simulink model "gtm_aeromodel"  (Simulink 7.2)
settings: Solver=ode45  StartTime=0.0  StopTime=10.0  RelTol=1e-3
undefined symbols (not defined in the file or in its folder): A_BLCG, A_BW, A_CW, A_FSCG, A_FSREF_in, A_SW, A_WLCG, A_WLREF, ALPHA0, bclowb, bclowbx_FMACH, bcmowb, bcmowbx_FHP, bcmowby_FMACH, cda, cdax_FLPDEF, cddr, cddrx_FMACH, cdo, cdox_FLPDEF, cdt1, cdt1x_mach, cdt2, cdt2x_mach, cdto, cdtox_mach, cdwb, cdwbx_FALPHA, cdwby_FMACH, clat, clatfr, clatfrx_FHP, clatfry_FMACH, clatx_mach, clawbfr, clawbfrx_FHP, clawbfry_FMACH, cldefr, cldefrx_FHP, cldefry_FMACH, cldtab, cldtabx_FMACH, clqwb, clqwbfr, clqwbfrx_FHP, clqwbfry_FMACH, clqwbx_mach, cltdd, cltddx_FHP, cltddy_FMACH, clwb, clwbtdd, clwbtddx_FHP, clwbtddy_FMACH, clwbx_FALPHA, clwby_FMACH, clwbzdd, clwbzddx_FHP, clwbzddy_FMACH, clzdd ... (+196)
libraries: model_lib x1
(part 9 of 10)

== system gtm_aeromodel/get aero forces and moments/AERODYNAMICS/Moment Coefficients/PITCH/CMWB/CMWBFLEX ==
  note: tddco2g=fqadot*fcbar/(2*32.174)
  altitude : Inport  OutDataType=sfix(16)  OutScaling=2^0
  Mach : Inport  Port=2  OutDataType=sfix(16)  OutScaling=2^0
  NZB g's : Inport  Port=3  OutDataType=sfix(16)  OutScaling=2^0
  qdot : Inport  Port=4  OutDataType=sfix(16)  OutScaling=2^0
  Enable : EnablePort
  Fcn1 : Fcn  Expr=1/u
  Product1 : Product  OutDataType=sfix(16)  OutScaling=2^0  SaturateOnIntegerOverflow=on  RndMeth=Zero  InputSameDT=on  OutDataTypeStr=Inherit: Same as first input
  Product2 : Product  Inputs=3  OutDataType=sfix(16)  OutScaling=2^0  SaturateOnIntegerOverflow=on  RndMeth=Zero  InputSameDT=on  OutDataTypeStr=Inherit: Same as first input
  Product3 : Product  OutDataType=sfix(16)  OutScaling=2^0  SaturateOnIntegerOverflow=on  RndMeth=Zero  InputSameDT=on  OutDataTypeStr=Inherit: Same as first input
  Product4 : Product  OutDataType=sfix(16)  OutScaling=2^0  SaturateOnIntegerOverflow=on  RndMeth=Zero  InputSameDT=on  OutDataTypeStr=Inherit: Same as first input
  Sum3 : Sum  OutDataType=sfix(16)  OutScaling=2^0  SaturateOnIntegerOverflow=on  InputSameDT=on  OutDataTypeStr=Inherit: Same as first input
  Wing Chord : Constant  Value=A_CW  OutDataType=sfix(16)  OutScaling=2^0
  Wing Chord1 : Constant  Value=2  OutDataType=sfix(16)  OutScaling=2^0
  Wing Chord2 : Constant  Value=constants.g  OutDataType=sfix(16)  OutScaling=2^0
  cmawbfr_ : Subsystem  mask(2-D Table){y=cmawbfrx_FHP, z=cmawbfry_FMACH, tab=cmawbfr}
      mask prompts: y "Y vector:"; z "Z vector:"; tab "Table:"
      mask help: 2-D Table Look Up. Enter monotonic Y and Z vectors and a matrix of 2-D tables. See the help for more info.
      mask Help: The Y and Z vectors must be monotonic.  Y  indexes into the columns of the 2-D table & Z indexes into the rows of the 2-D tables.   The input values are y and z respectively (e.g., top port = y).
      mask Display: plot(-10,-10,110,110,[90,50,10],[90,40,30],[90,50,10],[50,26,20],[90,50,10],[22,13,10])
  cmwbtdd : Subsystem  mask(2-D Table){y=cmwbtddx_FHP, z=cmwbtddy_FMACH, tab=cmwbtdd}
      mask prompts: y "Y vector:"; z "Z vector:"; tab "Table:"
      mask help: 2-D Table Look Up. Enter monotonic Y and Z vectors and a matrix of 2-D tables. See the help for more info.
      mask Help: The Y and Z vectors must be monotonic.  Y  indexes into the columns of the 2-D table & Z indexes into the rows of the 2-D tables.   The input values are y and z respectively (e.g., top port = y).
      mask Display: plot(-10,-10,110,110,[90,50,10],[90,40,30],[90,50,10],[50,26,20],[90,50,10],[22,13,10])
  cmwbzdd : Subsystem  mask(2-D Table){y=cmwbzddx_FHP, z=cmwbzddy_FMACH, tab=cmwbzdd}
      mask prompts: y "Y vector:"; z "Z vector:"; tab "Table:"
      mask help: 2-D Table Look Up. Enter monotonic Y and Z vectors and a matrix of 2-D tables. See the help for more info.
      mask Help: The Y and Z vectors must be monotonic.  Y  indexes into the columns of the 2-D table & Z indexes into the rows of the 2-D tables.   The input values are y and z respectively (e.g., top port = y).
      mask Display: plot(-10,-10,110,110,[90,50,10],[90,40,30],[90,50,10],[50,26,20],[90,50,10],[22,13,10])
  dcmowbflex_ : Subsystem  mask(2-D Table){y=dcmowbflexx_FHP, z=dcmowbflexy_FMACH, tab=dcmowbflex}
      mask prompts: y "Y vector:"; z "Z vector:"; tab "Table:"
      mask help: 2-D Table Look Up. Enter monotonic Y and Z vectors and a matrix of 2-D tables. See the help for more info.
      mask Help: The Y and Z vectors must be monotonic.  Y  indexes into the columns of the 2-D table & Z indexes into the rows of the 2-D tables.   The input values are y and z respectively (e.g., top port = y).
      mask Display: plot(-10,-10,110,110,[90,50,10],[90,40,30],[90,50,10],[50,26,20],[90,50,10],[22,13,10])
  cm_flx : Outport  OutDataType=sfix(16)  OutScaling=2^0  InitialOutput=0
  cmawbfr : Outport  Port=2  OutDataType=sfix(16)  OutScaling=2^0  InitialOutput=0
  fdcmowb : Outport  Port=3  OutDataType=sfix(16)  OutScaling=2^0  InitialOutput=0
  wires:
  cmwbzdd/1(Interp Value) -> Product1/1
  cmwbtdd/1(Interp Value) -> Product2/1
  Sum3/1 -> cm_flx/1
  Product1/1 -> Sum3/1
  dcmowbflex_/1(Interp Value) -> fdcmowb/1
  Wing Chord1/1 -> Product4/1
  Fcn1/1 -> Product2/3
  Product3/1 -> Product2/2
  qdot/1 -> Product3/1
  Product4/1 -> Fcn1/1
  Wing Chord2/1 -> Product4/2
  Wing Chord/1 -> Product3/2
  cmawbfr_/1(Interp Value) -> cmawbfr/1
  altitude/1 -> cmwbtdd/1(Y), cmwbzdd/1(Y), cmawbfr_/1(Y), dcmowbflex_/1(Y)
  Mach/1 -> cmwbtdd/2(Z), cmwbzdd/2(Z), cmawbfr_/2(Z), dcmowbflex_/2(Z)
  Product2/1 -> Sum3/2
  NZB g's/1 -> Product1/2

== system gtm_aeromodel/get aero forces and moments/AERODYNAMICS/Moment Coefficients/PITCH/CMWB/cm_flap_ ==
  flap : Inport  OutDataType=sfix(16)  OutScaling=2^0
  alpha : Inport  Port=2  OutDataType=sfix(16)  OutScaling=2^0
  qdyn : Inport  Port=3  OutDataType=sfix(16)  OutScaling=2^0
  flex : Inport  Port=4  OutDataType=sfix(16)  OutScaling=2^0
  dsb : Inport  Port=5  OutDataType=sfix(16)  OutScaling=2^0
  Enable : EnablePort
  DSB : Constant  Value=0.0  OutDataType=sfix(16)  OutScaling=2^0
  MACH : Constant  Value=0.178  OutDataType=sfix(16)  OutScaling=2^0
  Product : Product  OutDataType=sfix(16)  OutScaling=2^0  SaturateOnIntegerOverflow=on  RndMeth=Zero  InputSameDT=on  OutDataTypeStr=Inherit: Same as first input
  Sum : Sum  Inputs=+-  OutDataType=sfix(16)  OutScaling=2^0  SaturateOnIntegerOverflow=on  InputSameDT=on  OutDataTypeStr=Inherit: Same as first input
  Sum1 : Sum  Inputs=+--  OutDataType=sfix(16)  OutScaling=2^0  SaturateOnIntegerOverflow=on  InputSameDT=on  OutDataTypeStr=Inherit: Same as first input
  Switch5 : Switch  Threshold=0.5  SaturateOnIntegerOverflow=on  InputSameDT=on
  cmwb : Subsystem  mask(2-D Table){y=cmwbx_FALPHA, z=cmwby_FMACH, tab=cmwb}
      mask prompts: y "Y vector:"; z "Z vector:"; tab "Table:"
      mask help: 2-D Table Look Up. Enter monotonic Y and Z vectors and a matrix of 2-D tables. See the help for more info.
      mask Help: The Y and Z vectors must be monotonic.  Y  indexes into the columns of the 2-D table & Z indexes into the rows of the 2-D tables.   The input values are y and z respectively (e.g., top port = y).
      mask Display: plot(-10,-10,110,110,[90,50,10],[90,40,30],[90,50,10],[50,26,20],[90,50,10],[22,13,10])
  cmwbdsbdf : Subsystem  mask(1-2-3 Table){@1=cmwbdsbdfx_DSB, @2=cmwbdsbdfy_FALPHA, @3=cmwbdsbdfz_FLPDEF, @4=cmwbdsbdf}
      mask prompts: @1 "X vector:"; @2 "Y vector:"; @3 "Z vector:"; @4 "Table:"
      mask help: 3-D Table Look Up. Enter monotonic X, Y and Z vectors and a matrix of 2-D tables. See the help for more info.
      mask init:
      | x=@1;y=@2;z=@3;tab=@4;
      mask Help: The X, Y and Z vectors must be monotonic.   The 3-D table is a horizontal concatenation of  2-D tables.  X  indexes into the columns of the 2-D tables & Y indexes into the rows of the 2-D tables.  Z indexes into the table levels (starting with the 1st 2-D table).   The input values are x, y and z respectively (e.g., top port = x).
      mask Display: plot([0 2 2 0 0],[0 0 2 2 0],[0 2 2.9 0.95 0],[2 2 2.7 2.7 2],[2 2.9 2.9 2 2],[0 0.85 2.7 2 0])
  cmwbdsbdf1 : Subsystem  mask(1-2-3 Table){@1=cmwbdsbdfx_DSB, @2=cmwbdsbdfy_FALPHA, @3=cmwbdsbdfz_FLPDEF, @4=cmwbdsbdf}
      mask prompts: @1 "X vector:"; @2 "Y vector:"; @3 "Z vector:"; @4 "Table:"
      mask help: 3-D Table Look Up. Enter monotonic X, Y and Z vectors and a matrix of 2-D tables. See the help for more info.
      mask init:
      | x=@1;y=@2;z=@3;tab=@4;
      mask Help: The X, Y and Z vectors must be monotonic.   The 3-D table is a horizontal concatenation of  2-D tables.  X  indexes into the columns of the 2-D tables & Y indexes into the rows of the 2-D tables.  Z indexes into the table levels (starting with the 1st 2-D table).   The input values are x, y and z respectively (e.g., top port = x).
      mask Display: plot([0 2 2 0 0],[0 0 2 2 0],[0 2 2.9 0.95 0],[2 2 2.7 2.7 2],[2 2.9 2.9 2 2],[0 0.85 2.7 2 0])
  const : Constant  Value=1.0  OutDataType=sfix(16)  OutScaling=2^0
  dcmwbdffr : Subsystem  mask(2-D Table){y=dcmwbdffrx_FQ, z=dcmwbdffry_FLPDEF, tab=dcmwbdffr}
      mask prompts: y "Y vector:"; z "Z vector:"; tab "Table:"
      mask help: 2-D Table Look Up. Enter monotonic Y and Z vectors and a matrix of 2-D tables. See the help for more info.
      mask Help: The Y and Z vectors must be monotonic.  Y  indexes into the columns of the 2-D table & Z indexes into the rows of the 2-D tables.   The input values are y and z respectively (e.g., top port = y).
      mask Display: plot(-10,-10,110,110,[90,50,10],[90,40,30],[90,50,10],[50,26,20],[90,50,10],[22,13,10])
  dcmwbdsb : Subsystem  mask(1-2-3 Table){@1=dcmwbdsbx_DSB, @2=dcmwbdsby_ALPHA, @3=dcmwbdsbz_FMACH, @4=dcmwbdsb}
      mask prompts: @1 "X vector:"; @2 "Y vector:"; @3 "Z vector:"; @4 "Table:"
      mask help: 3-D Table Look Up. Enter monotonic X, Y and Z vectors and a matrix of 2-D tables. See the help for more info.
      mask init:
      | x=@1;y=@2;z=@3;tab=@4;
      mask Help: The X, Y and Z vectors must be monotonic.   The 3-D table is a horizontal concatenation of  2-D tables.  X  indexes into the columns of the 2-D tables & Y indexes into the rows of the 2-D tables.  Z indexes into the table levels (starting with the 1st 2-D table).   The input values are x, y and z respectively (e.g., top port = x).
      mask Display: plot([0 2 2 0 0],[0 0 2 2 0],[0 2 2.9 0.95 0],[2 2 2.7 2.7 2],[2 2.9 2.9 2 2],[0 0.85 2.7 2 0])
  cm_flap : Outport  OutDataType=sfix(16)  OutScaling=2^0  InitialOutput=0
  dcmsbfint : Outport  Port=2  OutDataType=sfix(16)  OutScaling=2^0  InitialOutput=0
  wires:
  Sum1/1 -> dcmsbfint/1
  dcmwbdffr/1(Interp Value) -> Switch5/1
  cmwbdsbdf/1(Interp Value) -> Sum1/2, Sum/1
  cmwbdsbdf1/1(Interp Value) -> Sum1/1
  Switch5/1 -> Product/2
  const/1 -> Switch5/3
  flex/1 -> Switch5/2
  qdyn/1 -> dcmwbdffr/1(Y)
  Product/1 -> cm_flap/1
  flap/1 -> cmwbdsbdf1/3(Z), dcmwbdffr/2(Z), cmwbdsbdf/3(Z)
  Sum/1 -> Product/1
  alpha/1 -> cmwbdsbdf/2(Y), cmwbdsbdf1/2(Y), dcmwbdsb/2(Y), cmwb/1(Y)
  DSB/1 -> cmwbdsbdf/1(X)
  dcmwbdsb/1(Interp Value) -> Sum1/3
  MACH/1 -> dcmwbdsb/3(Z), cmwb/2(Z)
  dsb/1 -> cmwbdsbdf1/1(X), dcmwbdsb/1(X)
  cmwb/1(Interp Value) -> Sum/2

== system gtm_aeromodel/get aero forces and moments/AERODYNAMICS/Moment Coefficients/PITCH/CMWB/cmwb_ ==
  Y : Inport  OutDataType=sfix(16)  OutScaling=2^0
  Z : Inport  Port=2  OutDataType=sfix(16)  OutScaling=2^0
  Mux : Mux  Inputs=2
  S-Function : S-Function  FunctionName=table2v5  Parameters=y,z,tab  EnableBusSupport=off
  Interp Value : Outport  OutDataType=sfix(16)  OutScaling=2^0
  wires:
  Mux/1 -> S-Function/1
  S-Function/1 -> Interp Value/1
  Y/1 -> Mux/1
  Z/1 -> Mux/2

== system gtm_aeromodel/get aero forces and moments/AERODYNAMICS/Moment Coefficients/PITCH/CMWB/cmwb_zero ==
  Y : Inport  OutDataType=sfix(16)  OutScaling=2^0
  Z : Inport  Port=2  OutDataType=sfix(16)  OutScaling=2^0
  Mux : Mux  Inputs=2
  S-Function : S-Function  FunctionName=table2v5  Parameters=y,z,tab  EnableBusSupport=off
  Interp Value : Outport  OutDataType=sfix(16)  OutScaling=2^0
  wires:
  Z/1 -> Mux/2
  Y/1 -> Mux/1
  S-Function/1 -> Interp Value/1
  Mux/1 -> S-Function/1

== system gtm_aeromodel/get aero forces and moments/AERODYNAMICS/Moment Coefficients/PITCH/DCMDE/cmdefr ==
  altitude : Inport  OutDataType=sfix(16)  OutScaling=2^0
  mach : Inport  Port=2  OutDataType=sfix(16)  OutScaling=2^0
  Enable : EnablePort
  cmdefr_ : Subsystem  mask(2-D Table){y=cmdefrx_FHP, z=cmdefry_FMACH, tab=cmdefr}
      mask prompts: y "Y vector:"; z "Z vector:"; tab "Table:"
      mask help: 2-D Table Look Up. Enter monotonic Y and Z vectors and a matrix of 2-D tables. See the help for more info.
      mask Help: The Y and Z vectors must be monotonic.  Y  indexes into the columns of the 2-D table & Z indexes into the rows of the 2-D tables.   The input values are y and z respectively (e.g., top port = y).
      mask Display: plot(-10,-10,110,110,[90,50,10],[90,40,30],[90,50,10],[50,26,20],[90,50,10],[22,13,10])
  cmdefr : Outport  OutDataType=sfix(16)  OutScaling=2^0  InitialOutput=0
  wires:
  mach/1 -> cmdefr_/2(Z)
  altitude/1 -> cmdefr_/1(Y)
  cmdefr_/1(Interp Value) -> cmdefr/1

== system gtm_aeromodel/get aero forces and moments/AERODYNAMICS/Moment Coefficients/PITCH/DCMDE/dcmde_ ==
  X : Inport  OutDataType=sfix(16)  OutScaling=2^0
  Y : Inport  Port=2  OutDataType=sfix(16)  OutScaling=2^0
  Z : Inport  Port=3  OutDataType=sfix(16)  OutScaling=2^0
  Mux : Mux  Inputs=3
  S-Function : S-Function  FunctionName=table3v5  Parameters=x,y,z,tab  EnableBusSupport=off
  Interp Value : Outport  OutDataType=sfix(16)  OutScaling=2^0
  wires:
  S-Function/1 -> Interp Value/1
  Mux/1 -> S-Function/1
  X/1 -> Mux/1
  Y/1 -> Mux/2
  Z/1 -> Mux/3

== system gtm_aeromodel/get aero forces and moments/AERODYNAMICS/Moment Coefficients/ROLL/CRAIL/CAILFLEX ==
  altitude : Inport  OutDataType=sfix(16)  OutScaling=2^0
  Mach : Inport  Port=2  OutDataType=sfix(16)  OutScaling=2^0
  Enable : EnablePort
  crdafr_ : Subsystem  mask(2-D Table){y=crdafrx_FHP, z=crdafry_FMACH, tab=crdafr}
      mask prompts: y "Y vector:"; z "Z vector:"; tab "Table:"
      mask help: 2-D Table Look Up. Enter monotonic Y and Z vectors and a matrix of 2-D tables. See the help for more info.
      mask Help: The Y and Z vectors must be monotonic.  Y  indexes into the columns of the 2-D table & Z indexes into the rows of the 2-D tables.   The input values are y and z respectively (e.g., top port = y).
      mask Display: plot(-10,-10,110,110,[90,50,10],[90,40,30],[90,50,10],[50,26,20],[90,50,10],[22,13,10])
  crdafr : Outport  OutDataType=sfix(16)  OutScaling=2^0  InitialOutput=0
  wires:
  altitude/1 -> crdafr_/1(Y)
  Mach/1 -> crdafr_/2(Z)
  crdafr_/1(Interp Value) -> crdafr/1

== system gtm_aeromodel/get aero forces and moments/AERODYNAMICS/Moment Coefficients/ROLL/CRAIL/crda ==
  X : Inport  OutDataType=sfix(16)  OutScaling=2^0
  Y : Inport  Port=2  OutDataType=sfix(16)  OutScaling=2^0
  Z : Inport  Port=3  OutDataType=sfix(16)  OutScaling=2^0
  Mux : Mux  Inputs=3
  S-Function : S-Function  FunctionName=table3v5  Parameters=x,y,z,tab  EnableBusSupport=off
  Interp Value : Outport  OutDataType=sfix(16)  OutScaling=2^0
  wires:
  Z/1 -> Mux/3
  Y/1 -> Mux/2
  X/1 -> Mux/1
  Mux/1 -> S-Function/1
  S-Function/1 -> Interp Value/1

== system gtm_aeromodel/get aero forces and moments/AERODYNAMICS/Moment Coefficients/ROLL/CRAIL/crda1 ==
  X : Inport  OutDataType=sfix(16)  OutScaling=2^0
  Y : Inport  Port=2  OutDataType=sfix(16)  OutScaling=2^0
  Z : Inport  Port=3  OutDataType=sfix(16)  OutScaling=2^0
  Mux : Mux  Inputs=3
  S-Function : S-Function  FunctionName=table3v5  Parameters=x,y,z,tab  EnableBusSupport=off
  Interp Value : Outport  OutDataType=sfix(16)  OutScaling=2^0
  wires:
  S-Function/1 -> Interp Value/1
  Mux/1 -> S-Function/1
  X/1 -> Mux/1
  Y/1 -> Mux/2
  Z/1 -> Mux/3

== system gtm_aeromodel/get aero forces and moments/AERODYNAMICS/Moment Coefficients/ROLL/CRAIL/crdadot ==
  Z : Inport  OutDataType=sfix(16)  OutScaling=2^0
  S-Function : S-Function  FunctionName=table1v5  Parameters=z,tab  EnableBusSupport=off
  Interp Value : Outport  OutDataType=sfix(16)  OutScaling=2^0
  wires:
  S-Function/1 -> Interp Value/1
  Z/1 -> S-Function/1

== system gtm_aeromodel/get aero forces and moments/AERODYNAMICS/Moment Coefficients/ROLL/CRAIL/crdadot1 ==
  Z : Inport  OutDataType=sfix(16)  OutScaling=2^0
  S-Function : S-Function  FunctionName=table1v5  Parameters=z,tab  EnableBusSupport=off
  Interp Value : Outport  OutDataType=sfix(16)  OutScaling=2^0
  wires:
  Z/1 -> S-Function/1
  S-Function/1 -> Interp Value/1

== system gtm_aeromodel/get aero forces and moments/AERODYNAMICS/Moment Coefficients/ROLL/CRBWB/CRWBFLEX ==
  altitude : Inport  OutDataType=sfix(16)  OutScaling=2^0
  Mach : Inport  Port=2  OutDataType=sfix(16)  OutScaling=2^0
  Enable : EnablePort
  crbfr_ : Subsystem  mask(2-D Table){y=crbfrx_FHP, z=crbfry_FMACH, tab=crbfr}
      mask prompts: y "Y vector:"; z "Z vector:"; tab "Table:"
      mask help: 2-D Table Look Up. Enter monotonic Y and Z vectors and a matrix of 2-D tables. See the help for more info.
      mask Help: The Y and Z vectors must be monotonic.  Y  indexes into the columns of the 2-D table & Z indexes into the rows of the 2-D tables.   The input values are y and z respectively (e.g., top port = y).
      mask Display: plot(-10,-10,110,110,[90,50,10],[90,40,30],[90,50,10],[50,26,20],[90,50,10],[22,13,10])
  crbfr : Outport  OutDataType=sfix(16)  OutScaling=2^0  InitialOutput=0
  wires:
  Mach/1 -> crbfr_/2(Z)
  altitude/1 -> crbfr_/1(Y)
  crbfr_/1(Interp Value) -> crbfr/1

== system gtm_aeromodel/get aero forces and moments/AERODYNAMICS/Moment Coefficients/ROLL/CRBWB/cr_flap_ ==
  flap : Inport  OutDataType=sfix(16)  OutScaling=2^0
  alpha : Inport  Port=2  OutDataType=sfix(16)  OutScaling=2^0
  Enable : EnablePort
  dcrbdf1 : Subsystem  mask(2-D Table){y=dcrbdfx_FLPDEF, z=dcrbdfy_FALPHA, tab=dcrbdf}
      mask prompts: y "Y vector:"; z "Z vector:"; tab "Table:"
      mask help: 2-D Table Look Up. Enter monotonic Y and Z vectors and a matrix of 2-D tables. See the help for more info.
      mask Help: The Y and Z vectors must be monotonic.  Y  indexes into the columns of the 2-D table & Z indexes into the rows of the 2-D tables.   The input values are y and z respectively (e.g., top port = y).
      mask Display: plot(-10,-10,110,110,[90,50,10],[90,40,30],[90,50,10],[50,26,20],[90,50,10],[22,13,10])
  cr_flap : Outport  OutDataType=sfix(16)  OutScaling=2^0  InitialOutput=0
  wires:
  flap/1 -> dcrbdf1/1(Y)
  alpha/1 -> dcrbdf1/2(Z)
  dcrbdf1/1(Interp Value) -> cr_flap/1

== system gtm_aeromodel/get aero forces and moments/AERODYNAMICS/Moment Coefficients/ROLL/CRBWB/crbwb_ ==
  Y : Inport  OutDataType=sfix(16)  OutScaling=2^0
  Z : Inport  Port=2  OutDataType=sfix(16)  OutScaling=2^0
  Mux : Mux  Inputs=2
  S-Function : S-Function  FunctionName=table2v5  Parameters=y,z,tab  EnableBusSupport=off
  Interp Value : Outport  OutDataType=sfix(16)  OutScaling=2^0
  wires:
  Z/1 -> Mux/2
  Y/1 -> Mux/1
  S-Function/1 -> Interp Value/1
  Mux/1 -> S-Function/1

== system gtm_aeromodel/get aero forces and moments/AERODYNAMICS/Moment Coefficients/ROLL/CRGEAR/dcrb_ ==
  Z : Inport  OutDataType=sfix(16)  OutScaling=2^0
  S-Function : S-Function  FunctionName=table1v5  Parameters=z,tab  EnableBusSupport=off
  Interp Value : Outport  OutDataType=sfix(16)  OutScaling=2^0
  wires:
  Z/1 -> S-Function/1
  S-Function/1 -> Interp Value/1

== system gtm_aeromodel/get aero forces and moments/AERODYNAMICS/Moment Coefficients/ROLL/CRP/CRPFLEX ==
  altitude : Inport  OutDataType=sfix(16)  OutScaling=2^0
  Mach : Inport  Port=2  OutDataType=sfix(16)  OutScaling=2^0
  Enable : EnablePort
  crpfr_ : Subsystem  mask(2-D Table){y=crpfrx_FHP, z=crpfry_FMACH, tab=crpfr}
      mask prompts: y "Y vector:"; z "Z vector:"; tab "Table:"
      mask help: 2-D Table Look Up. Enter monotonic Y and Z vectors and a matrix of 2-D tables. See the help for more info.
      mask Help: The Y and Z vectors must be monotonic.  Y  indexes into the columns of the 2-D table & Z indexes into the rows of the 2-D tables.   The input values are y and z respectively (e.g., top port = y).
      mask Display: plot(-10,-10,110,110,[90,50,10],[90,40,30],[90,50,10],[50,26,20],[90,50,10],[22,13,10])
  crpfr : Outport  OutDataType=sfix(16)  OutScaling=2^0  InitialOutput=0
  wires:
  Mach/1 -> crpfr_/2(Z)
  altitude/1 -> crpfr_/1(Y)
  crpfr_/1(Interp Value) -> crpfr/1

== system gtm_aeromodel/get aero forces and moments/AERODYNAMICS/Moment Coefficients/ROLL/CRP/crpwb_ ==
  Y : Inport  OutDataType=sfix(16)  OutScaling=2^0
  Z : Inport  Port=2  OutDataType=sfix(16)  OutScaling=2^0
  Mux : Mux  Inputs=2
  S-Function : S-Function  FunctionName=table2v5  Parameters=y,z,tab  EnableBusSupport=off
  Interp Value : Outport  OutDataType=sfix(16)  OutScaling=2^0
  wires:
  Z/1 -> Mux/2
  Y/1 -> Mux/1
  S-Function/1 -> Interp Value/1
  Mux/1 -> S-Function/1

== system gtm_aeromodel/get aero forces and moments/AERODYNAMICS/Moment Coefficients/ROLL/CRP/rcrbvt ==
  Y : Inport  OutDataType=sfix(16)  OutScaling=2^0
  Z : Inport  Port=2  OutDataType=sfix(16)  OutScaling=2^0
  Mux : Mux  Inputs=2
  S-Function : S-Function  FunctionName=table2v5  Parameters=y,z,tab  EnableBusSupport=off
  Interp Value : Outport  OutDataType=sfix(16)  OutScaling=2^0
  wires:
  Mux/1 -> S-Function/1
  S-Function/1 -> Interp Value/1
  Y/1 -> Mux/1
  Z/1 -> Mux/2

== system gtm_aeromodel/get aero forces and moments/AERODYNAMICS/Moment Coefficients/ROLL/CRP/rcybvt ==
  Y : Inport  OutDataType=sfix(16)  OutScaling=2^0
  Z : Inport  Port=2  OutDataType=sfix(16)  OutScaling=2^0
  Mux : Mux  Inputs=2
  S-Function : S-Function  FunctionName=table2v5  Parameters=y,z,tab  EnableBusSupport=off
  Interp Value : Outport  OutDataType=sfix(16)  OutScaling=2^0
  wires:
  Z/1 -> Mux/2
  Y/1 -> Mux/1
  S-Function/1 -> Interp Value/1
  Mux/1 -> S-Function/1

== system gtm_aeromodel/get aero forces and moments/AERODYNAMICS/Moment Coefficients/ROLL/CRR/CRRFLEX ==
  altitude : Inport  OutDataType=sfix(16)  OutScaling=2^0
  Mach : Inport  Port=2  OutDataType=sfix(16)  OutScaling=2^0
  Enable : EnablePort
  crrfr_ : Subsystem  mask(2-D Table){y=crrfrx_FHP, z=crrfry_FMACH, tab=crrfr}
      mask prompts: y "Y vector:"; z "Z vector:"; tab "Table:"
      mask help: 2-D Table Look Up. Enter monotonic Y and Z vectors and a matrix of 2-D tables. See the help for more info.
      mask Help: The Y and Z vectors must be monotonic.  Y  indexes into the columns of the 2-D table & Z indexes into the rows of the 2-D tables.   The input values are y and z respectively (e.g., top port = y).
      mask Display: plot(-10,-10,110,110,[90,50,10],[90,40,30],[90,50,10],[50,26,20],[90,50,10],[22,13,10])
  crrfr : Outport  OutDataType=sfix(16)  OutScaling=2^0  InitialOutput=0
  wires:
  altitude/1 -> crrfr_/1(Y)
  Mach/1 -> crrfr_/2(Z)
  crrfr_/1(Interp Value) -> crrfr/1

== system gtm_aeromodel/get aero forces and moments/AERODYNAMICS/Moment Coefficients/ROLL/CRR/crrwb_ ==
  Y : Inport  OutDataType=sfix(16)  OutScaling=2^0
  Z : Inport  Port=2  OutDataType=sfix(16)  OutScaling=2^0
  Mux : Mux  Inputs=2
  S-Function : S-Function  FunctionName=table2v5  Parameters=y,z,tab  EnableBusSupport=off
  Interp Value : Outport  OutDataType=sfix(16)  OutScaling=2^0
  wires:
  Z/1 -> Mux/2
  Y/1 -> Mux/1
  S-Function/1 -> Interp Value/1
  Mux/1 -> S-Function/1

== system gtm_aeromodel/get aero forces and moments/AERODYNAMICS/Moment Coefficients/ROLL/CRR/rcnbvt ==
  Y : Inport  OutDataType=sfix(16)  OutScaling=2^0
  Z : Inport  Port=2  OutDataType=sfix(16)  OutScaling=2^0
  Mux : Mux  Inputs=2
  S-Function : S-Function  FunctionName=table2v5  Parameters=y,z,tab  EnableBusSupport=off
  Interp Value : Outport  OutDataType=sfix(16)  OutScaling=2^0
  wires:
  Mux/1 -> S-Function/1
  S-Function/1 -> Interp Value/1
  Y/1 -> Mux/1
  Z/1 -> Mux/2

== system gtm_aeromodel/get aero forces and moments/AERODYNAMICS/Moment Coefficients/ROLL/CRR/rcrbvt ==
  Y : Inport  OutDataType=sfix(16)  OutScaling=2^0
  Z : Inport  Port=2  OutDataType=sfix(16)  OutScaling=2^0
  Mux : Mux  Inputs=2
  S-Function : S-Function  FunctionName=table2v5  Parameters=y,z,tab  EnableBusSupport=off
  Interp Value : Outport  OutDataType=sfix(16)  OutScaling=2^0
  wires:
  Mux/1 -> S-Function/1
  S-Function/1 -> Interp Value/1
  Y/1 -> Mux/1
  Z/1 -> Mux/2

== system gtm_aeromodel/get aero forces and moments/AERODYNAMICS/Moment Coefficients/ROLL/CRR/rcybvt ==
  Y : Inport  OutDataType=sfix(16)  OutScaling=2^0
  Z : Inport  Port=2  OutDataType=sfix(16)  OutScaling=2^0
  Mux : Mux  Inputs=2
  S-Function : S-Function  FunctionName=table2v5  Parameters=y,z,tab  EnableBusSupport=off
  Interp Value : Outport  OutDataType=sfix(16)  OutScaling=2^0
  wires:
  Z/1 -> Mux/2
  Y/1 -> Mux/1
  S-Function/1 -> Interp Value/1
  Mux/1 -> S-Function/1

== system gtm_aeromodel/get aero forces and moments/AERODYNAMICS/Moment Coefficients/ROLL/CRRUD/CRFLEX ==
  altitude : Inport  OutDataType=sfix(16)  OutScaling=2^0
  Mach : Inport  Port=2  OutDataType=sfix(16)  OutScaling=2^0
  Enable : EnablePort
  crdrfr2 : Subsystem  mask(2-D Table){y=crdrfrx_FHP, z=crdrfry_FMACH, tab=crdrfr}
      mask prompts: y "Y vector:"; z "Z vector:"; tab "Table:"
      mask help: 2-D Table Look Up. Enter monotonic Y and Z vectors and a matrix of 2-D tables. See the help for more info.
      mask Help: The Y and Z vectors must be monotonic.  Y  indexes into the columns of the 2-D table & Z indexes into the rows of the 2-D tables.   The input values are y and z respectively (e.g., top port = y).
      mask Display: plot(-10,-10,110,110,[90,50,10],[90,40,30],[90,50,10],[50,26,20],[90,50,10],[22,13,10])
  crdrfr : Outport  OutDataType=sfix(16)  OutScaling=2^0  InitialOutput=0
  wires:
  crdrfr2/1(Interp Value) -> crdrfr/1
  altitude/1 -> crdrfr2/1(Y)
  Mach/1 -> crdrfr2/2(Z)

== system gtm_aeromodel/get aero forces and moments/AERODYNAMICS/Moment Coefficients/ROLL/CRRUD/crdr ==
  Z : Inport  OutDataType=sfix(16)  OutScaling=2^0
  S-Function : S-Function  FunctionName=table1v5  Parameters=z,tab  EnableBusSupport=off
  Interp Value : Outport  OutDataType=sfix(16)  OutScaling=2^0
  wires:
  S-Function/1 -> Interp Value/1
  Z/1 -> S-Function/1

== system gtm_aeromodel/get aero forces and moments/AERODYNAMICS/Moment Coefficients/ROLL/CRSPOIL/cr_sp_fl ==
  flap : Inport  OutDataType=sfix(16)  OutScaling=2^0
  alpha : Inport  Port=2  OutDataType=sfix(16)  OutScaling=2^0
  dsl : Inport  Port=3  OutDataType=sfix(16)  OutScaling=2^0
  dsb : Inport  Port=4  OutDataType=sfix(16)  OutScaling=2^0
  dsr : Inport  Port=5  OutDataType=sfix(16)  OutScaling=2^0
  Enable : EnablePort
  Sum1 : Sum  Inputs=+-  OutDataType=sfix(16)  OutScaling=2^0  SaturateOnIntegerOverflow=on  InputSameDT=on  OutDataTypeStr=Inherit: Same as first input
  Sum2 : Sum  Inputs=+-  OutDataType=sfix(16)  OutScaling=2^0  SaturateOnIntegerOverflow=on  InputSameDT=on  OutDataTypeStr=Inherit: Same as first input
  Sum3 : Sum  Inputs=+-  OutDataType=sfix(16)  OutScaling=2^0  SaturateOnIntegerOverflow=on  InputSameDT=on  OutDataTypeStr=Inherit: Same as first input
  dcrwbdsldf : Subsystem  mask(1-2-3 Table){@1=dcrwbdsldfx_DSL, @2=dcrwbdsldfy_FALPHA, @3=dcrwbdsldfz_FLPDEF, @4=dcrwbdsldf}
      mask prompts: @1 "X vector:"; @2 "Y vector:"; @3 "Z vector:"; @4 "Table:"
      mask help: 3-D Table Look Up. Enter monotonic X, Y and Z vectors and a matrix of 2-D tables. See the help for more info.
      mask init:
      | x=@1;y=@2;z=@3;tab=@4;
      mask Help: The X, Y and Z vectors must be monotonic.   The 3-D table is a horizontal concatenation of  2-D tables.  X  indexes into the columns of the 2-D tables & Y indexes into the rows of the 2-D tables.  Z indexes into the table levels (starting with the 1st 2-D table).   The input values are x, y and z respectively (e.g., top port = x).
      mask Display: plot([0 2 2 0 0],[0 0 2 2 0],[0 2 2.9 0.95 0],[2 2 2.7 2.7 2],[2 2.9 2.9 2 2],[0 0.85 2.7 2 0])
  dcrwbdsldf1 : Subsystem  mask(1-2-3 Table){@1=dcrwbdsldfx_DSL, @2=dcrwbdsldfy_FALPHA, @3=dcrwbdsldfz_FLPDEF, @4=dcrwbdsldf}
      mask prompts: @1 "X vector:"; @2 "Y vector:"; @3 "Z vector:"; @4 "Table:"
      mask help: 3-D Table Look Up. Enter monotonic X, Y and Z vectors and a matrix of 2-D tables. See the help for more info.
      mask init:
      | x=@1;y=@2;z=@3;tab=@4;
      mask Help: The X, Y and Z vectors must be monotonic.   The 3-D table is a horizontal concatenation of  2-D tables.  X  indexes into the columns of the 2-D tables & Y indexes into the rows of the 2-D tables.  Z indexes into the table levels (starting with the 1st 2-D table).   The input values are x, y and z respectively (e.g., top port = x).
      mask Display: plot([0 2 2 0 0],[0 0 2 2 0],[0 2 2.9 0.95 0],[2 2 2.7 2.7 2],[2 2.9 2.9 2 2],[0 0.85 2.7 2 0])
  dcrwbdsldf2 : Subsystem  mask(1-2-3 Table){@1=dcrwbdsldfx_DSL, @2=dcrwbdsldfy_FALPHA, @3=dcrwbdsldfz_FLPDEF, @4=dcrwbdsldf}
      mask prompts: @1 "X vector:"; @2 "Y vector:"; @3 "Z vector:"; @4 "Table:"
      mask help: 3-D Table Look Up. Enter monotonic X, Y and Z vectors and a matrix of 2-D tables. See the help for more info.
      mask init:
      | x=@1;y=@2;z=@3;tab=@4;
      mask Help: The X, Y and Z vectors must be monotonic.   The 3-D table is a horizontal concatenation of  2-D tables.  X  indexes into the columns of the 2-D tables & Y indexes into the rows of the 2-D tables.  Z indexes into the table levels (starting with the 1st 2-D table).   The input values are x, y and z respectively (e.g., top port = x).
      mask Display: plot([0 2 2 0 0],[0 0 2 2 0],[0 2 2.9 0.95 0],[2 2 2.7 2.7 2],[2 2.9 2.9 2 2],[0 0.85 2.7 2 0])
  cr_sp_fl : Outport  OutDataType=sfix(16)  OutScaling=2^0  InitialOutput=0
  wires:
  alpha/1 -> dcrwbdsldf/2(Y), dcrwbdsldf1/2(Y), dcrwbdsldf2/2(Y)
  dsl/1 -> dcrwbdsldf/1(X)
  dsb/1 -> dcrwbdsldf1/1(X)
  flap/1 -> dcrwbdsldf/3(Z), dcrwbdsldf1/3(Z), dcrwbdsldf2/3(Z)
  dcrwbdsldf/1(Interp Value) -> Sum1/1
  dsr/1 -> dcrwbdsldf2/1(X)
  dcrwbdsldf2/1(Interp Value) -> Sum2/1
  dcrwbdsldf1/1(Interp Value) -> Sum1/2, Sum2/2
  Sum1/1 -> Sum3/1
  Sum2/1 -> Sum3/2
  Sum3/1 -> cr_sp_fl/1

== system gtm_aeromodel/get aero forces and moments/AERODYNAMICS/Moment Coefficients/ROLL/CRSPOIL/cr_sp_flex ==
  altitude : Inport  OutDataType=sfix(16)  OutScaling=2^0
  mach : Inport  Port=2  OutDataType=sfix(16)  OutScaling=2^0
  Enable : EnablePort
  dcrdslfr : Subsystem  mask(2-D Table){y=dcrdslfrx_FHP, z=dcrdslfry_FMACH, tab=dcrdslfr}
      mask prompts: y "Y vector:"; z "Z vector:"; tab "Table:"
      mask help: 2-D Table Look Up. Enter monotonic Y and Z vectors and a matrix of 2-D tables. See the help for more info.
      mask Help: The Y and Z vectors must be monotonic.  Y  indexes into the columns of the 2-D table & Z indexes into the rows of the 2-D tables.   The input values are y and z respectively (e.g., top port = y).
      mask Display: plot(-10,-10,110,110,[90,50,10],[90,40,30],[90,50,10],[50,26,20],[90,50,10],[22,13,10])
  cr_sp_flex : Outport  OutDataType=sfix(16)  OutScaling=2^0  InitialOutput=0
  wires:
  dcrdslfr/1(Interp Value) -> cr_sp_flex/1
  mach/1 -> dcrdslfr/2(Z)
  altitude/1 -> dcrdslfr/1(Y)

== system gtm_aeromodel/get aero forces and moments/AERODYNAMICS/Moment Coefficients/ROLL/CRSPOIL/dcrwbdsbp ==
  X : Inport  OutDataType=sfix(16)  OutScaling=2^0
  Y : Inport  Port=2  OutDataType=sfix(16)  OutScaling=2^0
  Z : Inport  Port=3  OutDataType=sfix(16)  OutScaling=2^0
  Mux : Mux  Inputs=3
  S-Function : S-Function  FunctionName=table3v5  Parameters=x,y,z,tab  EnableBusSupport=off
  Interp Value : Outport  OutDataType=sfix(16)  OutScaling=2^0
  wires:
  Z/1 -> Mux/3
  Y/1 -> Mux/2
  X/1 -> Mux/1
  Mux/1 -> S-Function/1
  S-Function/1 -> Interp Value/1

== system gtm_aeromodel/get aero forces and moments/AERODYNAMICS/Moment Coefficients/ROLL/CRSPOIL/dcrwbdsl ==
  X : Inport  OutDataType=sfix(16)  OutScaling=2^0
  Y : Inport  Port=2  OutDataType=sfix(16)  OutScaling=2^0
  Z : Inport  Port=3  OutDataType=sfix(16)  OutScaling=2^0
  Mux : Mux  Inputs=3
  S-Function : S-Function  FunctionName=table3v5  Parameters=x,y,z,tab  EnableBusSupport=off
  Interp Value : Outport  OutDataType=sfix(16)  OutScaling=2^0
  wires:
  S-Function/1 -> Interp Value/1
  Mux/1 -> S-Function/1
  X/1 -> Mux/1
  Y/1 -> Mux/2
  Z/1 -> Mux/3

== system gtm_aeromodel/get aero forces and moments/AERODYNAMICS/Moment Coefficients/ROLL/CRSPOIL/dcrwbdsl1 ==
  X : Inport  OutDataType=sfix(16)  OutScaling=2^0
  Y : Inport  Port=2  OutDataType=sfix(16)  OutScaling=2^0
  Z : Inport  Port=3  OutDataType=sfix(16)  OutScaling=2^0
  Mux : Mux  Inputs=3
  S-Function : S-Function  FunctionName=table3v5  Parameters=x,y,z,tab  EnableBusSupport=off
  Interp Value : Outport  OutDataType=sfix(16)  OutScaling=2^0
  wires:
  Z/1 -> Mux/3
  Y/1 -> Mux/2
  X/1 -> Mux/1
  Mux/1 -> S-Function/1
  S-Function/1 -> Interp Value/1

== system gtm_aeromodel/get aero forces and moments/AERODYNAMICS/Moment Coefficients/ROLL/CRSPOIL/dcrwbdsl2 ==
  X : Inport  OutDataType=sfix(16)  OutScaling=2^0
  Y : Inport  Port=2  OutDataType=sfix(16)  OutScaling=2^0
  Z : Inport  Port=3  OutDataType=sfix(16)  OutScaling=2^0
  Mux : Mux  Inputs=3
  S-Function : S-Function  FunctionName=table3v5  Parameters=x,y,z,tab  EnableBusSupport=off
  Interp Value : Outport  OutDataType=sfix(16)  OutScaling=2^0
  wires:
  S-Function/1 -> Interp Value/1
  Mux/1 -> S-Function/1
  X/1 -> Mux/1
  Y/1 -> Mux/2
  Z/1 -> Mux/3

== system gtm_aeromodel/get aero forces and moments/AERODYNAMICS/Moment Coefficients/ROLL/CRSPOIL/dcrwbdsl3 ==
  X : Inport  OutDataType=sfix(16)  OutScaling=2^0
  Y : Inport  Port=2  OutDataType=sfix(16)  OutScaling=2^0
  Z : Inport  Port=3  OutDataType=sfix(16)  OutScaling=2^0
  Mux : Mux  Inputs=3
  S-Function : S-Function  FunctionName=table3v5  Parameters=x,y,z,tab  EnableBusSupport=off
  Interp Value : Outport  OutDataType=sfix(16)  OutScaling=2^0
  wires:
  Z/1 -> Mux/3
  Y/1 -> Mux/2
  X/1 -> Mux/1
  Mux/1 -> S-Function/1
  S-Function/1 -> Interp Value/1

== system gtm_aeromodel/get aero forces and moments/AERODYNAMICS/Moment Coefficients/ROLL/CRSPOIL/dcrwbdsl4 ==
  X : Inport  OutDataType=sfix(16)  OutScaling=2^0
  Y : Inport  Port=2  OutDataType=sfix(16)  OutScaling=2^0
  Z : Inport  Port=3  OutDataType=sfix(16)  OutScaling=2^0
  Mux : Mux  Inputs=3
  S-Function : S-Function  FunctionName=table3v5  Parameters=x,y,z,tab  EnableBusSupport=off
  Interp Value : Outport  OutDataType=sfix(16)  OutScaling=2^0
  wires:
  S-Function/1 -> Interp Value/1
  Mux/1 -> S-Function/1
  X/1 -> Mux/1
  Y/1 -> Mux/2
  Z/1 -> Mux/3

== system gtm_aeromodel/get aero forces and moments/AERODYNAMICS/Moment Coefficients/ROLL/TAIL/crbht ==
  Y : Inport  OutDataType=sfix(16)  OutScaling=2^0
  Z : Inport  Port=2  OutDataType=sfix(16)  OutScaling=2^0
  Mux : Mux  Inputs=2
  S-Function : S-Function  FunctionName=table2v5  Parameters=y,z,tab  EnableBusSupport=off
  Interp Value : Outport  OutDataType=sfix(16)  OutScaling=2^0
  wires:
  Z/1 -> Mux/2
  Y/1 -> Mux/1
  S-Function/1 -> Interp Value/1
  Mux/1 -> S-Function/1

== system gtm_aeromodel/get aero forces and moments/AERODYNAMICS/Moment Coefficients/ROLL/TAIL/crbvt ==
  Y : Inport  OutDataType=sfix(16)  OutScaling=2^0
  Z : Inport  Port=2  OutDataType=sfix(16)  OutScaling=2^0
  Mux : Mux  Inputs=2
  S-Function : S-Function  FunctionName=table2v5  Parameters=y,z,tab  EnableBusSupport=off
  Interp Value : Outport  OutDataType=sfix(16)  OutScaling=2^0
  wires:
  Z/1 -> Mux/2
  Y/1 -> Mux/1
  S-Function/1 -> Interp Value/1
  Mux/1 -> S-Function/1

== system gtm_aeromodel/get aero forces and moments/AERODYNAMICS/Moment Coefficients/YAW/CNBWB/CNWBFLEX ==
  altitude : Inport  OutDataType=sfix(16)  OutScaling=2^0
  Mach : Inport  Port=2  OutDataType=sfix(16)  OutScaling=2^0
  Enable : EnablePort
  cnbfr_ : Subsystem  mask(2-D Table){y=cnbfrx_FHP, z=cnbfry_FMACH, tab=cnbfr}
      mask prompts: y "Y vector:"; z "Z vector:"; tab "Table:"
      mask help: 2-D Table Look Up. Enter monotonic Y and Z vectors and a matrix of 2-D tables. See the help for more info.
      mask Help: The Y and Z vectors must be monotonic.  Y  indexes into the columns of the 2-D table & Z indexes into the rows of the 2-D tables.   The input values are y and z respectively (e.g., top port = y).
      mask Display: plot(-10,-10,110,110,[90,50,10],[90,40,30],[90,50,10],[50,26,20],[90,50,10],[22,13,10])
  cnbfr : Outport  OutDataType=sfix(16)  OutScaling=2^0  InitialOutput=0
  wires:
  cnbfr_/1(Interp Value) -> cnbfr/1
  altitude/1 -> cnbfr_/1(Y)
  Mach/1 -> cnbfr_/2(Z)

== system gtm_aeromodel/get aero forces and moments/AERODYNAMICS/Moment Coefficients/YAW/CNBWB/cn_flap_ ==
  flap : Inport  OutDataType=sfix(16)  OutScaling=2^0
  alpha : Inport  Port=2  OutDataType=sfix(16)  OutScaling=2^0
  Enable : EnablePort
  dcnbdf : Subsystem  mask(2-D Table){y=dcnbdfx_FLPDEF, z=dcnbdfy_FALPHA, tab=dcnbdf}
      mask prompts: y "Y vector:"; z "Z vector:"; tab "Table:"
      mask help: 2-D Table Look Up. Enter monotonic Y and Z vectors and a matrix of 2-D tables. See the help for more info.
      mask Help: The Y and Z vectors must be monotonic.  Y  indexes into the columns of the 2-D table & Z indexes into the rows of the 2-D tables.   The input values are y and z respectively (e.g., top port = y).
      mask Display: plot(-10,-10,110,110,[90,50,10],[90,40,30],[90,50,10],[50,26,20],[90,50,10],[22,13,10])
  cn_flap : Outport  OutDataType=sfix(16)  OutScaling=2^0  InitialOutput=0
  wires:
  alpha/1 -> dcnbdf/2(Z)
  flap/1 -> dcnbdf/1(Y)
  dcnbdf/1(Interp Value) -> cn_flap/1

== system gtm_aeromodel/get aero forces and moments/AERODYNAMICS/Moment Coefficients/YAW/CNBWB/cnbwb_ ==
  Y : Inport  OutDataType=sfix(16)  OutScaling=2^0
  Z : Inport  Port=2  OutDataType=sfix(16)  OutScaling=2^0
  Mux : Mux  Inputs=2
  S-Function : S-Function  FunctionName=table2v5  Parameters=y,z,tab  EnableBusSupport=off
  Interp Value : Outport  OutDataType=sfix(16)  OutScaling=2^0
  wires:
  Z/1 -> Mux/2
  Y/1 -> Mux/1
  S-Function/1 -> Interp Value/1
  Mux/1 -> S-Function/1

== system gtm_aeromodel/get aero forces and moments/AERODYNAMICS/Moment Coefficients/YAW/CNGEAR/dcnb ==
  Z : Inport  OutDataType=sfix(16)  OutScaling=2^0
  S-Function : S-Function  FunctionName=table1v5  Parameters=z,tab  EnableBusSupport=off
  Interp Value : Outport  OutDataType=sfix(16)  OutScaling=2^0
  wires:
  S-Function/1 -> Interp Value/1
  Z/1 -> S-Function/1

== system gtm_aeromodel/get aero forces and moments/AERODYNAMICS/Moment Coefficients/YAW/CNP/CNPFLEX ==
  altitude : Inport  OutDataType=sfix(16)  OutScaling=2^0
  Mach : Inport  Port=2  OutDataType=sfix(16)  OutScaling=2^0
  Enable : EnablePort
  cnpfr_ : Subsystem  mask(2-D Table){y=cnpfrx_FHP, z=cnpfry_FMACH, tab=cnpfr}
      mask prompts: y "Y vector:"; z "Z vector:"; tab "Table:"
      mask help: 2-D Table Look Up. Enter monotonic Y and Z vectors and a matrix of 2-D tables. See the help for more info.
      mask Help: The Y and Z vectors must be monotonic.  Y  indexes into the columns of the 2-D table & Z indexes into the rows of the 2-D tables.   The input values are y and z respectively (e.g., top port = y).
      mask Display: plot(-10,-10,110,110,[90,50,10],[90,40,30],[90,50,10],[50,26,20],[90,50,10],[22,13,10])
  cnpfr : Outport  OutDataType=sfix(16)  OutScaling=2^0  InitialOutput=0
  wires:
  altitude/1 -> cnpfr_/1(Y)
  Mach/1 -> cnpfr_/2(Z)
  cnpfr_/1(Interp Value) -> cnpfr/1

== system gtm_aeromodel/get aero forces and moments/AERODYNAMICS/Moment Coefficients/YAW/CNP/rcnbvt ==
  Y : Inport  OutDataType=sfix(16)  OutScaling=2^0
  Z : Inport  Port=2  OutDataType=sfix(16)  OutScaling=2^0
  Mux : Mux  Inputs=2
  S-Function : S-Function  FunctionName=table2v5  Parameters=y,z,tab  EnableBusSupport=off
  Interp Value : Outport  OutDataType=sfix(16)  OutScaling=2^0
  wires:
  Z/1 -> Mux/2
  Y/1 -> Mux/1
  S-Function/1 -> Interp Value/1
  Mux/1 -> S-Function/1

== system gtm_aeromodel/get aero forces and moments/AERODYNAMICS/Moment Coefficients/YAW/CNP/rcnpwb ==
  Y : Inport  OutDataType=sfix(16)  OutScaling=2^0
  Z : Inport  Port=2  OutDataType=sfix(16)  OutScaling=2^0
  Mux : Mux  Inputs=2
  S-Function : S-Function  FunctionName=table2v5  Parameters=y,z,tab  EnableBusSupport=off
  Interp Value : Outport  OutDataType=sfix(16)  OutScaling=2^0
  wires:
  Z/1 -> Mux/2
  Y/1 -> Mux/1
  S-Function/1 -> Interp Value/1
  Mux/1 -> S-Function/1

== system gtm_aeromodel/get aero forces and moments/AERODYNAMICS/Moment Coefficients/YAW/CNP/rcrbvt ==
  Y : Inport  OutDataType=sfix(16)  OutScaling=2^0
  Z : Inport  Port=2  OutDataType=sfix(16)  OutScaling=2^0
  Mux : Mux  Inputs=2
  S-Function : S-Function  FunctionName=table2v5  Parameters=y,z,tab  EnableBusSupport=off
  Interp Value : Outport  OutDataType=sfix(16)  OutScaling=2^0
  wires:
  Z/1 -> Mux/2
  Y/1 -> Mux/1
  S-Function/1 -> Interp Value/1
  Mux/1 -> S-Function/1

== system gtm_aeromodel/get aero forces and moments/AERODYNAMICS/Moment Coefficients/YAW/CNP/rcybvt ==
  Y : Inport  OutDataType=sfix(16)  OutScaling=2^0
  Z : Inport  Port=2  OutDataType=sfix(16)  OutScaling=2^0
  Mux : Mux  Inputs=2
  S-Function : S-Function  FunctionName=table2v5  Parameters=y,z,tab  EnableBusSupport=off
  Interp Value : Outport  OutDataType=sfix(16)  OutScaling=2^0
  wires:
  Mux/1 -> S-Function/1
  S-Function/1 -> Interp Value/1
  Y/1 -> Mux/1
  Z/1 -> Mux/2

== system gtm_aeromodel/get aero forces and moments/AERODYNAMICS/Moment Coefficients/YAW/CNR/CNRFLEX ==
  altitude : Inport  OutDataType=sfix(16)  OutScaling=2^0
  Mach : Inport  Port=2  OutDataType=sfix(16)  OutScaling=2^0
  Enable : EnablePort
  cnrfr_ : Subsystem  mask(2-D Table){y=cnrfrx_FHP, z=cnrfry_FMACH, tab=cnrfr}
      mask prompts: y "Y vector:"; z "Z vector:"; tab "Table:"
      mask help: 2-D Table Look Up. Enter monotonic Y and Z vectors and a matrix of 2-D tables. See the help for more info.
      mask Help: The Y and Z vectors must be monotonic.  Y  indexes into the columns of the 2-D table & Z indexes into the rows of the 2-D tables.   The input values are y and z respectively (e.g., top port = y).
      mask Display: plot(-10,-10,110,110,[90,50,10],[90,40,30],[90,50,10],[50,26,20],[90,50,10],[22,13,10])
  cnrfr : Outport  OutDataType=sfix(16)  OutScaling=2^0  InitialOutput=0
  wires:
  Mach/1 -> cnrfr_/2(Z)
  altitude/1 -> cnrfr_/1(Y)
  cnrfr_/1(Interp Value) -> cnrfr/1

== system gtm_aeromodel/get aero forces and moments/AERODYNAMICS/Moment Coefficients/YAW/CNR/rcnbvt ==
  Y : Inport  OutDataType=sfix(16)  OutScaling=2^0
  Z : Inport  Port=2  OutDataType=sfix(16)  OutScaling=2^0
  Mux : Mux  Inputs=2
  S-Function : S-Function  FunctionName=table2v5  Parameters=y,z,tab  EnableBusSupport=off
  Interp Value : Outport  OutDataType=sfix(16)  OutScaling=2^0
  wires:
  Z/1 -> Mux/2
  Y/1 -> Mux/1
  S-Function/1 -> Interp Value/1
  Mux/1 -> S-Function/1

== system gtm_aeromodel/get aero forces and moments/AERODYNAMICS/Moment Coefficients/YAW/CNR/rcnrwb ==
  Y : Inport  OutDataType=sfix(16)  OutScaling=2^0
  Z : Inport  Port=2  OutDataType=sfix(16)  OutScaling=2^0
  Mux : Mux  Inputs=2
  S-Function : S-Function  FunctionName=table2v5  Parameters=y,z,tab  EnableBusSupport=off
  Interp Value : Outport  OutDataType=sfix(16)  OutScaling=2^0
  wires:
  Z/1 -> Mux/2
  Y/1 -> Mux/1
  S-Function/1 -> Interp Value/1
  Mux/1 -> S-Function/1

== system gtm_aeromodel/get aero forces and moments/AERODYNAMICS/Moment Coefficients/YAW/CNR/rcybvt ==
  Y : Inport  OutDataType=sfix(16)  OutScaling=2^0
  Z : Inport  Port=2  OutDataType=sfix(16)  OutScaling=2^0
  Mux : Mux  Inputs=2
  S-Function : S-Function  FunctionName=table2v5  Parameters=y,z,tab  EnableBusSupport=off
  Interp Value : Outport  OutDataType=sfix(16)  OutScaling=2^0
  wires:
  Mux/1 -> S-Function/1
  S-Function/1 -> Interp Value/1
  Y/1 -> Mux/1
  Z/1 -> Mux/2

== system gtm_aeromodel/get aero forces and moments/AERODYNAMICS/Moment Coefficients/YAW/CNRUD/CNFLEX ==
  altitude : Inport  OutDataType=sfix(16)  OutScaling=2^0
  Mach : Inport  Port=2  OutDataType=sfix(16)  OutScaling=2^0
  Enable : EnablePort
  cndrfr_ : Subsystem  mask(2-D Table){y=cndrfrx_FHP, z=cndrfry_FMACH, tab=cndrfr}
      mask prompts: y "Y vector:"; z "Z vector:"; tab "Table:"
      mask help: 2-D Table Look Up. Enter monotonic Y and Z vectors and a matrix of 2-D tables. See the help for more info.
      mask Help: The Y and Z vectors must be monotonic.  Y  indexes into the columns of the 2-D table & Z indexes into the rows of the 2-D tables.   The input values are y and z respectively (e.g., top port = y).
      mask Display: plot(-10,-10,110,110,[90,50,10],[90,40,30],[90,50,10],[50,26,20],[90,50,10],[22,13,10])
  cndrfr : Outport  OutDataType=sfix(16)  OutScaling=2^0  InitialOutput=0
  wires:
  Mach/1 -> cndrfr_/2(Z)
  altitude/1 -> cndrfr_/1(Y)
  cndrfr_/1(Interp Value) -> cndrfr/1

== system gtm_aeromodel/get aero forces and moments/AERODYNAMICS/Moment Coefficients/YAW/CNRUD/cndr ==
  Z : Inport  OutDataType=sfix(16)  OutScaling=2^0
  S-Function : S-Function  FunctionName=table1v5  Parameters=z,tab  EnableBusSupport=off
  Interp Value : Outport  OutDataType=sfix(16)  OutScaling=2^0
  wires:
  S-Function/1 -> Interp Value/1
  Z/1 -> S-Function/1

== system gtm_aeromodel/get aero forces and moments/AERODYNAMICS/Moment Coefficients/YAW/CNSPOIL/cn_sp_fl ==
  flap : Inport  OutDataType=sfix(16)  OutScaling=2^0
  alpha : Inport  Port=2  OutDataType=sfix(16)  OutScaling=2^0
  dsl : Inport  Port=3  OutDataType=sfix(16)  OutScaling=2^0
  dsb : Inport  Port=4  OutDataType=sfix(16)  OutScaling=2^0
  dsr : Inport  Port=5  OutDataType=sfix(16)  OutScaling=2^0
  Enable : EnablePort
  Sum1 : Sum  Inputs=+-  OutDataType=sfix(16)  OutScaling=2^0  SaturateOnIntegerOverflow=on  InputSameDT=on  OutDataTypeStr=Inherit: Same as first input
  Sum2 : Sum  Inputs=+-  OutDataType=sfix(16)  OutScaling=2^0  SaturateOnIntegerOverflow=on  InputSameDT=on  OutDataTypeStr=Inherit: Same as first input
  Sum3 : Sum  Inputs=+-  OutDataType=sfix(16)  OutScaling=2^0  SaturateOnIntegerOverflow=on  InputSameDT=on  OutDataTypeStr=Inherit: Same as first input
  dcnwbdsldf : Subsystem  mask(1-2-3 Table){@1=dcnwbdsldfx_DSL, @2=dcnwbdsldfy_FALPHA, @3=dcnwbdsldfz_FLPDEF, @4=dcnwbdsldf}
      mask prompts: @1 "X vector:"; @2 "Y vector:"; @3 "Z vector:"; @4 "Table:"
      mask help: 3-D Table Look Up. Enter monotonic X, Y and Z vectors and a matrix of 2-D tables. See the help for more info.
      mask init:
      | x=@1;y=@2;z=@3;tab=@4;
      mask Help: The X, Y and Z vectors must be monotonic.   The 3-D table is a horizontal concatenation of  2-D tables.  X  indexes into the columns of the 2-D tables & Y indexes into the rows of the 2-D tables.  Z indexes into the table levels (starting with the 1st 2-D table).   The input values are x, y and z respectively (e.g., top port = x).
      mask Display: plot([0 2 2 0 0],[0 0 2 2 0],[0 2 2.9 0.95 0],[2 2 2.7 2.7 2],[2 2.9 2.9 2 2],[0 0.85 2.7 2 0])
  dcnwbdsldf1 : Subsystem  mask(1-2-3 Table){@1=dcnwbdsldfx_DSL, @2=dcnwbdsldfy_FALPHA, @3=dcnwbdsldfz_FLPDEF, @4=dcnwbdsldf}
      mask prompts: @1 "X vector:"; @2 "Y vector:"; @3 "Z vector:"; @4 "Table:"
      mask help: 3-D Table Look Up. Enter monotonic X, Y and Z vectors and a matrix of 2-D tables. See the help for more info.
      mask init:
      | x=@1;y=@2;z=@3;tab=@4;
      mask Help: The X, Y and Z vectors must be monotonic.   The 3-D table is a horizontal concatenation of  2-D tables.  X  indexes into the columns of the 2-D tables & Y indexes into the rows of the 2-D tables.  Z indexes into the table levels (starting with the 1st 2-D table).   The input values are x, y and z respectively (e.g., top port = x).
      mask Display: plot([0 2 2 0 0],[0 0 2 2 0],[0 2 2.9 0.95 0],[2 2 2.7 2.7 2],[2 2.9 2.9 2 2],[0 0.85 2.7 2 0])
  dcnwbdsldf2 : Subsystem  mask(1-2-3 Table){@1=dcnwbdsldfx_DSL, @2=dcnwbdsldfy_FALPHA, @3=dcnwbdsldfz_FLPDEF, @4=dcnwbdsldf}
      mask prompts: @1 "X vector:"; @2 "Y vector:"; @3 "Z vector:"; @4 "Table:"
      mask help: 3-D Table Look Up. Enter monotonic X, Y and Z vectors and a matrix of 2-D tables. See the help for more info.
      mask init:
      | x=@1;y=@2;z=@3;tab=@4;
      mask Help: The X, Y and Z vectors must be monotonic.   The 3-D table is a horizontal concatenation of  2-D tables.  X  indexes into the columns of the 2-D tables & Y indexes into the rows of the 2-D tables.  Z indexes into the table levels (starting with the 1st 2-D table).   The input values are x, y and z respectively (e.g., top port = x).
      mask Display: plot([0 2 2 0 0],[0 0 2 2 0],[0 2 2.9 0.95 0],[2 2 2.7 2.7 2],[2 2.9 2.9 2 2],[0 0.85 2.7 2 0])
  cn_sp_fl : Outport  OutDataType=sfix(16)  OutScaling=2^0  InitialOutput=0
  wires:
  Sum3/1 -> cn_sp_fl/1
  Sum2/1 -> Sum3/2
  Sum1/1 -> Sum3/1
  dcnwbdsldf1/1(Interp Value) -> Sum2/2, Sum1/2
  dcnwbdsldf2/1(Interp Value) -> Sum2/1
  dsr/1 -> dcnwbdsldf2/1(X)
  dcnwbdsldf/1(Interp Value) -> Sum1/1
  flap/1 -> dcnwbdsldf2/3(Z), dcnwbdsldf1/3(Z), dcnwbdsldf/3(Z)
  dsb/1 -> dcnwbdsldf1/1(X)
  dsl/1 -> dcnwbdsldf/1(X)
  alpha/1 -> dcnwbdsldf2/2(Y), dcnwbdsldf1/2(Y), dcnwbdsldf/2(Y)

== system gtm_aeromodel/get aero forces and moments/AERODYNAMICS/Moment Coefficients/YAW/CNSPOIL/dcnwbdsl ==
  X : Inport  OutDataType=sfix(16)  OutScaling=2^0
  Y : Inport  Port=2  OutDataType=sfix(16)  OutScaling=2^0
  Z : Inport  Port=3  OutDataType=sfix(16)  OutScaling=2^0
  Mux : Mux  Inputs=3
  S-Function : S-Function  FunctionName=table3v5  Parameters=x,y,z,tab  EnableBusSupport=off
  Interp Value : Outport  OutDataType=sfix(16)  OutScaling=2^0
  wires:
  S-Function/1 -> Interp Value/1
  Mux/1 -> S-Function/1
  X/1 -> Mux/1
  Y/1 -> Mux/2
  Z/1 -> Mux/3

== system gtm_aeromodel/get aero forces and moments/AERODYNAMICS/Moment Coefficients/YAW/CNSPOIL/dcnwbdsl1 ==
  X : Inport  OutDataType=sfix(16)  OutScaling=2^0
  Y : Inport  Port=2  OutDataType=sfix(16)  OutScaling=2^0
  Z : Inport  Port=3  OutDataType=sfix(16)  OutScaling=2^0
  Mux : Mux  Inputs=3
  S-Function : S-Function  FunctionName=table3v5  Parameters=x,y,z,tab  EnableBusSupport=off
  Interp Value : Outport  OutDataType=sfix(16)  OutScaling=2^0
  wires:
  Z/1 -> Mux/3
  Y/1 -> Mux/2
  X/1 -> Mux/1
  Mux/1 -> S-Function/1
  S-Function/1 -> Interp Value/1

== system gtm_aeromodel/get aero forces and moments/AERODYNAMICS/Moment Coefficients/YAW/CNSPOIL/dcnwbdsl2 ==
  X : Inport  OutDataType=sfix(16)  OutScaling=2^0
  Y : Inport  Port=2  OutDataType=sfix(16)  OutScaling=2^0
  Z : Inport  Port=3  OutDataType=sfix(16)  OutScaling=2^0
  Mux : Mux  Inputs=3
  S-Function : S-Function  FunctionName=table3v5  Parameters=x,y,z,tab  EnableBusSupport=off
  Interp Value : Outport  OutDataType=sfix(16)  OutScaling=2^0
  wires:
  Z/1 -> Mux/3
  Y/1 -> Mux/2
  X/1 -> Mux/1
  Mux/1 -> S-Function/1
  S-Function/1 -> Interp Value/1
